simulink model "rev1BB"  (R2021a)
settings: Solver=FixedStepAuto  StartTime=0.0  StopTime=((((preLen+100+dataLenSymbols)*1+pad_first*3)*basePer))*2.5  RelTol=1e-3
values from neighbouring files (symbols this model uses):
  agcDesired = 0    [rev1BB_setup.m]
  agcStep = 2^-8    (= 0.00390625)    [rev1BB_setup.m]
  awgnSeed = abs(dBSnrRange(dBSnrInd)*1000+trial+10000000)    [plotBer.m]    (also in plotBerParSim.m; rev1BB_startup.m = 67)
  basePer = 1/baseFreq    (= 5e-08)    [rev1BB_setup.m]
  bitsPerSymbolHeader = log2(radixHeader)    [rev1BB_setup.m]
  bitsPerSymbolMax = log2(radixMax)    [rev1BB_setup.m]
  cefEarlyWarning = 256    [rev1BB_setup.m]
  cefLen = length(x_CEF)    [rev1BB_setup.m]
  cfoNcoWordLen = 16    [rev1BB_setup.m]
  channelFIR = zeros(1, round(maxSampleDelay)+1)    [rev1BB_simParams_setup.m]
  corr_peak_exclude_trigger = 1+corr_peak_trigger    (= 1.4)    [rev1BB_setup.m]
  corr_peak_trigger = 0.40    (= 0.4)    [rev1BB_setup.m]
  cr_i = 0.020    (= 0.02)    [rev1BB_setup.m]
  cr_i_preamp = 2^-9    (= 0.001953125)    [rev1BB_setup.m]
  cr_p = 0.015    [rev1BB_setup.m]
  dataLenSymbols = header_len_bytes*8/bitsPerSymbolHeader + frame_len_bytes*8/bitsPerSymbol    [rev1BB_setup.m]
  enableTRFreqCorrection = true    [rev1BB_setup.m]
  freeze_agc_in_CEF = true    [rev1BB_setup.m]
  freeze_agc_in_HeaderPayload = true    [rev1BB_setup.m]
  freeze_fineCFO_in_CEF = false    [rev1BB_setup.m]
  freeze_fineCFO_in_HeaderPayload = false    [rev1BB_setup.m]
  golay_type = golayType    (= 32)    [rev1BB_setup.m]
  golayType = 32    [rev1BB_setup.m]
  lmsEqDepth = 16    [rev1BB_setup.m]
  lmsStep_meta = (lmsStep_final - lmsStep_init)/cefLen    [rev1BB_setup.m]
  manChan = false    [rev1BB_simParams_setup.m]
  minSTFPeaks = 3    [rev1BB_setup.m]
  modBPS = [1, 2, 4]    [rev1BB_setup.m]
  modKeys = [0, 1, 2]    [rev1BB_setup.m]
  overSample = 3    [berCurve.m]    (also in rev1BB_setup.m = 4)
  qam16_demod_scale_factor = qam16_hdl_distance/qam16_power_normalized_distance    [rev1BB_setup.m]
  rcRxFilt = rcSqrtFilt    [rev1BB_setup.m]
  rcTxFilt = rcSqrtFilt    [rev1BB_setup.m]
  RxAGCCorrectionLoopPartition = 3    [rev1BB_setup.m]
  RxAGCPwrAvgPartition = 2    [rev1BB_setup.m]
  RxCoarseCFOPartition = 13    [rev1BB_setup.m]
  RxDemodPartition = 15    [rev1BB_setup.m]
  RxEQPartition = 14    [rev1BB_setup.m]
  RxFeedbackPipelining = 64*16    (= 1024)    [rev1BB_setup.m]
  RxFineCFOPartition = 15    [rev1BB_setup.m]
  RxFreezeControllerPartition = 17    [rev1BB_setup.m]
  RxFreezeFeedbackPipelining = RxFeedbackPipelining    (= 1024)    [rev1BB_setup.m]
  RxHeaderDemodPartition = 15    [rev1BB_setup.m]
  RxHeaderParsePartition = 15    [rev1BB_setup.m]
  RxPackerPartition = 16    [rev1BB_setup.m]
  RxPacketControllerPartition = 17    [rev1BB_setup.m]
  RxRRCPartition = 1    [rev1BB_setup.m]
  RxTimingRecoveryControlPartition = 8    [rev1BB_setup.m]
  RxTimingRecoveryDelayAccumPartition = 10    [rev1BB_setup.m]
  RxTimingRecoveryEarlyLatePartition = 10    [rev1BB_setup.m]
  RxTimingRecoveryFreqEstPartition = 10    [rev1BB_setup.m]
  RxTimingRecoveryGolayCorrelatorPartition = 6    [rev1BB_setup.m]
  RxTimingRecoveryGolayPeakDetectPartition = 7    [rev1BB_setup.m]
  RxTimingRecoverySymbolClockPartition = 9    [rev1BB_setup.m]
  RxTimingRecoveryVariableDelayPartition = 5    [rev1BB_setup.m]
  timing_cefEarlyWarningTollerance = 5    [rev1BB_setup.m]
  timing_correlator_pipeline = 1    [rev1BB_setup.m]
  timing_differentiator_grpDelay_roundUp = ceil((timing_differentiator_len)/2+timing_differentiator_pipeline)    [rev1BB_setup.m]
  timing_differentiator_pipeline = 1    [rev1BB_setup.m]
  timing_p = -0.215    [rev1BB_setup.m]
  timing_tolerance = 4    [rev1BB_setup.m]
  timingDifferentiatorFilt = timingDifferentiatorFiltObj.Coefficients    [rev1BB_setup.m]
  timingMaxSymbols = dataLenSymbols + length(x_CEF) + length(x_STF)/x_STFRepCount*2+100    [rev1BB_setup.m]
  timingRecoveryDoneSamplesEarly = floor(RxFeedbackPipelining/overSample) - delayToOutputFromDataFSM-1    [rev1BB_setup.m]
  timingRecoveryFreqCorrectionAvgLen = 32    [rev1BB_setup.m]
  timingRecoveryFreqCorrectionDiscardLastN = 2    [rev1BB_setup.m]
  trEarlyLateIGain = -0.000000050    (= -5e-08)    [rev1BB_setup.m]
  trEarlyLatePGain = -0.00225    [rev1BB_setup.m]
  trFarrowTaps = 4    [rev1BB_setup.m]
  trFeedbackPipelining = 64*8    (= 512)    [rev1BB_setup.m]
  trIntPhaseCounterInit = mod(timing_differentiator_grpDelay_roundUp, overSample)    [rev1BB_setup.m]
  trMatch = mod(-trLenToFSM, overSample)    [rev1BB_setup.m]
  trTappedDelayLen = trTappedDelayBase+trFarrowTaps    (= 44)    [rev1BB_setup.m]
  tx_rx_gain = 1    [rev1BB_simParams_setup.m]
  TxResampleModulatorPartition = 1    [rev1BB_setup.m]
  TxRRCFilterPartition = 2    [rev1BB_setup.m]
  txTimingOffset = 0    [plotBer.m]    (also in plotBerParSim.m; rev1BB_startup.m = 2e-05)
  txTimingPhase = channelizerUpDownSampling*overSample*4+1    [rev1BB_simParams_setup.m]
  x_CEF = xSpectrum_CEF_short    [rev1BB_setup.m]
  x_STFRepCount = nSpectrum_STFRepCount_short    (= 60)    [rev1BB_setup.m]
undefined symbols (not defined in the file or in its folder): doppler, magnitude
libraries: simulink x29, rev1CyclopsLib x20, commdigbbndpm3 x9, dspsigops x6, commdigbbndam3 x4, hdlsllib x2, commchan3 x2, commrflib2 x1
(part 1 of 3)
settings Model: Creator=cyarp  LastModifiedBy=cyarp
settings SolverCC: AlgebraicLoopSolver=TrustRegion
settings OptimizationCC: SimCompilerOptimization=on
settings DebuggingCC: SFMachineParentedDataDiag=warning
settings SFSimCC: SimHardwareAcceleration=native

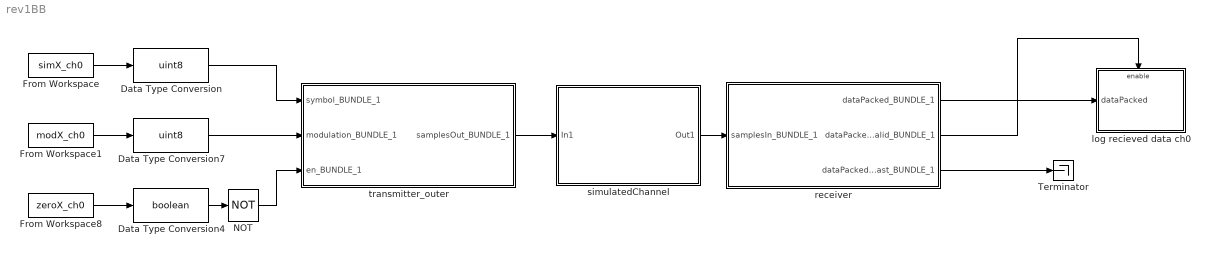
== system rev1BB ==
  Data Type Conversion : DataTypeConversion  OutDataTypeStr=uint8  RndMeth=Nearest
  Data Type Conversion4 : DataTypeConversion  OutDataTypeStr=boolean  RndMeth=Nearest
  Data Type Conversion7 : DataTypeConversion  OutDataTypeStr=uint8  RndMeth=Nearest
  From Workspace : FromWorkspace  VariableName=simX_ch0  SampleTime=basePer*1  Interpolate=off  OutputAfterFinalValue=Setting to zero
  From Workspace1 : FromWorkspace  VariableName=modX_ch0  SampleTime=basePer*1  Interpolate=off  OutputAfterFinalValue=Setting to zero
  From Workspace8 : FromWorkspace  VariableName=zeroX_ch0  SampleTime=basePer*1  Interpolate=off  OutputAfterFinalValue=Setting to zero
  NOT : Logic  Operator=NOT  IconShape=distinctive  AllPortsSameDT=off  OutDataTypeStr=boolean
  Terminator : Terminator
  log recieved data ch0 : Subsystem
  receiver : Subsystem
  simulatedChannel : Subsystem
  transmitter_outer : Subsystem
  wires:
  From Workspace/1 -> Data Type Conversion/1
  From Workspace1/1 -> Data Type Conversion7/1
  From Workspace8/1 -> Data Type Conversion4/1
  Data Type Conversion4/1 -> NOT/1
  simulatedChannel/1(Out1) -> receiver/1(samplesIn_BUNDLE_1)
  receiver/1(dataPacked_BUNDLE_1) -> log recieved data ch0/1(dataPacked)
  receiver/2(dataPackedValid_BUNDLE_1) -> log recieved data ch0/Enable
  receiver/3(dataPackedLast_BUNDLE_1) -> Terminator/1
  Data Type Conversion/1 -> transmitter_outer/1(symbol_BUNDLE_1)
  Data Type Conversion7/1 -> transmitter_outer/2(modulation_BUNDLE_1)
  NOT/1 -> transmitter_outer/3(en_BUNDLE_1)
  transmitter_outer/1(samplesOut_BUNDLE_1) -> simulatedChannel/1(In1)

== system rev1BB/log recieved data ch0 ==
  dataPacked : Inport
  Enable : EnablePort
  To Workspace1 : ToWorkspace  VariableName=data_recieved_packed_ch0  SampleTime=-1
      settings: Save2DSignal=2-D array (concatenate along first dimension)
  wires:
  dataPacked/1 -> To Workspace1/1

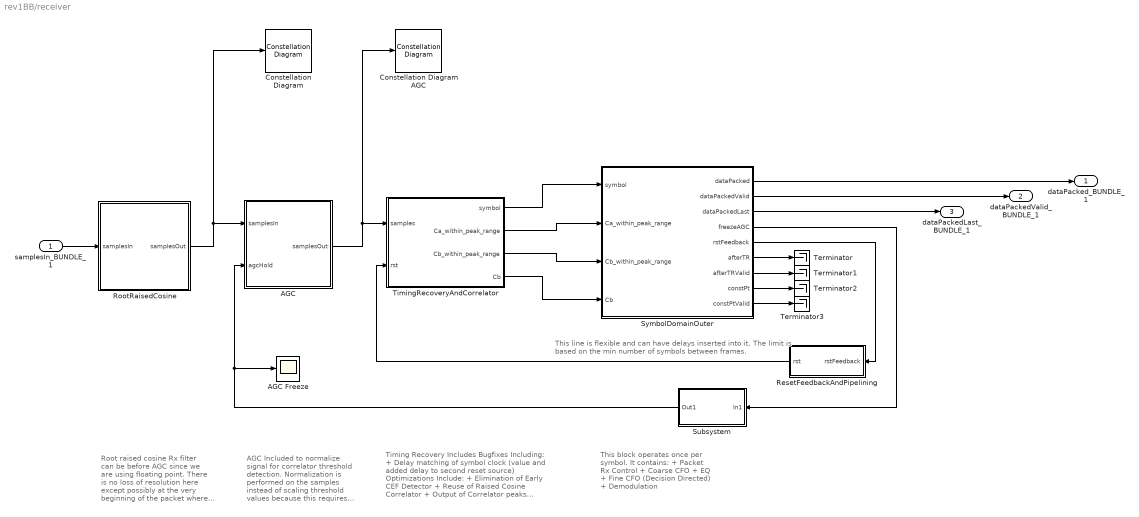
== system rev1BB/receiver ==
  note: This line is flexible and can have delays inserted into it.
      | The limit is based on the min number of symbols between frames.
  note: Timing Recovery Includes Bugfixes Including:
      | + Delay matching of symbol clock (value and added delay
      | to second reset source)
      |
      | Optimizations Include:
      | + Elimination of Early CEF Detector
      | + Reuse of Raised Cosine Correlator
      | + Output of Correlator peaks aligned with symbols
  note: This block operates once per symbol.
      |
      | It contains:
      | + Packet Rx Control
      | + Coarse CFO
      | + EQ
      | + Fine CFO (Decision Directed)
      | + Demodulation
  note: AGC Included to normalize signal for correlator threshold detection.  Normalization is performed on the samples instead of scaling threshold values because this requires fewer operations (once per sample instead of once per sample per threshold detector)
      |
      | This was also modified so that freezing the AGC stops power estimation.
  note: Root raised cosine Rx filter can be before AGC since we are using floating point. There is no loss of resolution here except possibly at the very beginning of the packet where a high power signal will show up.
  samplesIn_BUNDLE_1 : Inport
  AGC : Subsystem
  AGC Freeze : Scope
  Constellation Diagram : ConstellationDiagram
  Constellation Diagram AGC : ConstellationDiagram
  ResetFeedbackAndPipelining : Subsystem
  RootRaisedCosine : Subsystem
  Subsystem : Subsystem
  SymbolDomainOuter : Subsystem
  Terminator{,1..3} (4 alike) : Terminator
  TimingRecoveryAndCorrelator : Subsystem
  dataPacked_BUNDLE_1 : Outport
  dataPackedValid_BUNDLE_1 : Outport  Port=2
  dataPackedLast_BUNDLE_1 : Outport  Port=3
  wires:
  samplesIn_BUNDLE_1/1 -> RootRaisedCosine/1(samplesIn)
  AGC/1(samplesOut) -> Constellation Diagram AGC/1, TimingRecoveryAndCorrelator/1(samples)
  RootRaisedCosine/1(samplesOut) -> Constellation Diagram/1, AGC/1(samplesIn)
  ResetFeedbackAndPipelining/1(rst) -> TimingRecoveryAndCorrelator/2(rst)
  Subsystem/1(Out1) -> AGC Freeze/1, AGC/2(agcHold)
  TimingRecoveryAndCorrelator/1(symbol) -> SymbolDomainOuter/1(symbol)
  TimingRecoveryAndCorrelator/2(Ca_within_peak_range) -> SymbolDomainOuter/2(Ca_within_peak_range)
  TimingRecoveryAndCorrelator/3(Cb_within_peak_range) -> SymbolDomainOuter/3(Cb_within_peak_range)
  TimingRecoveryAndCorrelator/4(Cb) -> SymbolDomainOuter/4(Cb)
  SymbolDomainOuter/1(dataPacked) -> dataPacked_BUNDLE_1/1
  SymbolDomainOuter/2(dataPackedValid) -> dataPackedValid_BUNDLE_1/1
  SymbolDomainOuter/3(dataPackedLast) -> dataPackedLast_BUNDLE_1/1
  SymbolDomainOuter/4(freezeAGC) -> Subsystem/1(In1)
  SymbolDomainOuter/5(rstFeedback) -> ResetFeedbackAndPipelining/1(rstFeedback)
  SymbolDomainOuter/6(afterTR) -> Terminator/1
  SymbolDomainOuter/7(afterTRValid) -> Terminator1/1
  SymbolDomainOuter/8(constPt) -> Terminator2/1
  SymbolDomainOuter/9(constPtValid) -> Terminator3/1

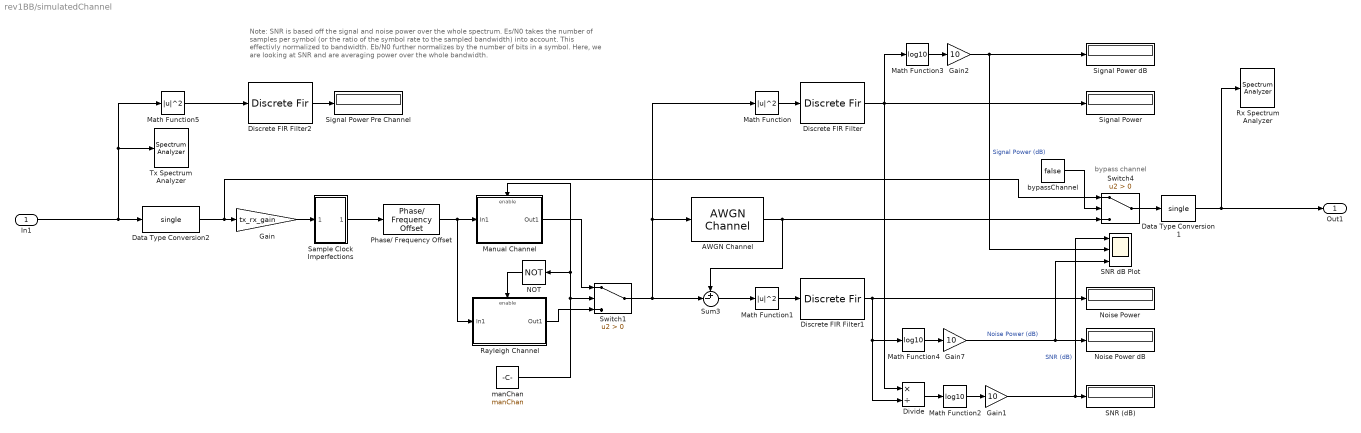
== system rev1BB/simulatedChannel ==
  note: Note: SNR is based off the signal and noise power over the whole spectrum.
      | Es/N0 takes the number of samples per symbol (or the ratio of the symbol rate to the sampled bandwidth) into account.  This effectivly normalized to bandwidth.
      | Eb/N0 further normalizes by the number of bits in a symbol.
      |
      | Here, we are looking at SNR and are averaging power over the whole bandwidth.
  note: bypass channel
  In1 : Inport
  AWGN Channel : commchan3/AWGN Channel  InputProcessing=Columns as channels (frame based)  seed=awgnSeed  noiseMode="Signal to noise ratio  (SNR)"  EbNodB=awgnEbN0  EsNodB=10  SNRdB=awgnSNR  bitsPerSym=1  Ps=1  Tsym=basePer  variance=1
  Data Type Conversion1 : DataTypeConversion  OutDataTypeStr=single
  Data Type Conversion2 : DataTypeConversion  OutDataTypeStr=single
  Discrete FIR Filter : DiscreteFir  Coefficients=ones(1,10000)./10000  InputProcessing=Columns as channels (frame based)
  Discrete FIR Filter1 : DiscreteFir  Coefficients=ones(1,10000)./10000  InputProcessing=Columns as channels (frame based)
  Discrete FIR Filter2 : DiscreteFir  Coefficients=ones(1,10000)./10000  InputProcessing=Columns as channels (frame based)
  Divide : Product  Inputs=*/
  Gain : Gain  Gain=tx_rx_gain
  Gain1 : Gain  Gain=10
  Gain2 : Gain  Gain=10
  Gain7 : Gain  Gain=10
  Manual Channel : Subsystem
  Math Function : Math  Operator=magnitude^2  SignedPower=on  OutputSignalType=real  SaturateOnIntegerOverflow=on
  Math Function1 : Math  Operator=magnitude^2  SignedPower=on  OutputSignalType=real  SaturateOnIntegerOverflow=on
  Math Function2 : Math  Operator=log10  SignedPower=on  OutputSignalType=real  SaturateOnIntegerOverflow=on
  Math Function3 : Math  Operator=log10  SignedPower=on  OutputSignalType=real  SaturateOnIntegerOverflow=on
  Math Function4 : Math  Operator=log10  SignedPower=on  OutputSignalType=real  SaturateOnIntegerOverflow=on
  Math Function5 : Math  Operator=magnitude^2  SignedPower=on  OutputSignalType=real  SaturateOnIntegerOverflow=on
  NOT : Logic  Operator=NOT  IconShape=distinctive  AllPortsSameDT=off  OutDataTypeStr=boolean
  Noise Power : Display
  Noise Power dB : Display
  Phase/ Frequency Offset : commrflib2/Phase// Frequency Offset  phaseOffset=rxPhaseOffset  freqPort=off  freqOffset=freqOffsetHz
  Rayleigh Channel : Subsystem
  Rx Spectrum Analyzer : SpectrumAnalyzer
  SNR (dB) : Display
  SNR dB Plot : Scope  NumInputPorts=3
  Sample Clock Imperfections : Subsystem
  Signal Power : Display
  Signal Power Pre Channel : Display
  Signal Power dB : Display
  Sum3 : Sum  Inputs=+-|
  Switch1 : Switch  Criteria=u2 > Threshold
  Switch4 : Switch  Criteria=u2 > Threshold
  Tx Spectrum Analyzer : SpectrumAnalyzer
  bypassChannel : Constant  Value=false  OutDataTypeStr=boolean
  manChan : Constant  Value=manChan  OutDataTypeStr=boolean
  Out1 : Outport
  wires:
  Data Type Conversion2/1 -> Switch4/1, Gain/1
  Sample Clock Imperfections/1(Out1) -> Phase/ Frequency Offset/1
  Data Type Conversion1/1 -> Out1/1, Rx Spectrum Analyzer/1
  bypassChannel/1 -> Switch4/2
  Gain2/1 -> SNR dB Plot/2, Signal Power dB/1  "Signal Power (dB)"
  AWGN Channel/1 -> Switch4/3, Sum3/1
  Gain/1 -> Sample Clock Imperfections/1(In1)
  Math Function/1 -> Discrete FIR Filter/1
  Sum3/1 -> Math Function1/1
  Switch1/1 -> Math Function/1, AWGN Channel/1, Sum3/2
  Math Function3/1 -> Gain2/1
  Gain7/1 -> SNR dB Plot/3, Noise Power dB/1  "Noise Power (dB)"
  Switch4/1 -> Data Type Conversion1/1
  Divide/1 -> Math Function2/1
  Gain1/1 -> SNR dB Plot/1, SNR (dB)/1  "SNR (dB)"
  Math Function2/1 -> Gain1/1
  Discrete FIR Filter/1 -> Math Function3/1, Divide/1, Signal Power/1
  Math Function4/1 -> Gain7/1
  Phase/ Frequency Offset/1 -> Manual Channel/1(In1), Rayleigh Channel/1(In1)
  Discrete FIR Filter1/1 -> Math Function4/1, Divide/2, Noise Power/1
  Math Function1/1 -> Discrete FIR Filter1/1
  In1/1 -> Math Function5/1, Tx Spectrum Analyzer/1, Data Type Conversion2/1
  Math Function5/1 -> Discrete FIR Filter2/1
  Discrete FIR Filter2/1 -> Signal Power Pre Channel/1
  manChan/1 -> Switch1/2, Manual Channel/Enable, NOT/1
  Rayleigh Channel/1(Out1) -> Switch1/3
  Manual Channel/1(Out1) -> Switch1/1
  NOT/1 -> Rayleigh Channel/Enable

== system rev1BB/transmitter_outer ==
  symbol_BUNDLE_1 : Inport
  modulation_BUNDLE_1 : Inport  Port=2
  en_BUNDLE_1 : Inport  Port=3
  transmitter : Subsystem
  samplesOut_BUNDLE_1 : Outport
  wires:
  transmitter/1(samplesOut) -> samplesOut_BUNDLE_1/1
  modulation_BUNDLE_1/1 -> transmitter/2(modulation)
  symbol_BUNDLE_1/1 -> transmitter/1(symbol)
  en_BUNDLE_1/1 -> transmitter/3(en)

== system rev1BB/receiver/AGC ==
  note: Note, the enabled subsystem was split because lazy FIFO evaluation
      | is not yet implemented in Laminar.  Because the enabled subsystems are all
      | driven by a common source and no state was placed between them,
      | the result should be the same.  Enabled subsystem is passed through the local
      | pipelines of partitions to hopefully capaitalize on communication locality
      | among these partitions (assuming these will be placed in the same L3).  Involves
      | using a dummy node to pass the enable signal in AGCLoopAndCorrect.
      |
      | Note that this arragment will cause one element to be in the sample FIFO into
      | AGCLoopAndCorrect at all times because of the dependence on AGC Pwr Avg
      |
      | ---
      | Change: Now forwarding samples from AGC Pwr Avg to AGCLoopAndCorrect.
  samplesIn : Inport
  agcHold : Inport  Port=2
  AGCLoopAndCorrect : Subsystem
  AGCPwrAvg : Subsystem
  Terminator : Terminator
  Terminator1 : Terminator
  samplesOut : Outport
  wires:
  samplesIn/1 -> AGCPwrAvg/1(samples)
  agcHold/1 -> AGCPwrAvg/2(freeze)
  AGCPwrAvg/2(lnPwrAvg) -> AGCLoopAndCorrect/2(pwrAvg)
  AGCPwrAvg/3(en) -> AGCLoopAndCorrect/3(enable)
  AGCLoopAndCorrect/1(samplesOut) -> samplesOut/1
  AGCPwrAvg/1(samplesOut) -> AGCLoopAndCorrect/1(samplesIn)
  AGCLoopAndCorrect/2(lnPwr) -> Terminator/1
  AGCLoopAndCorrect/3(en) -> Terminator1/1

== system rev1BB/receiver/ResetFeedbackAndPipelining ==
  rstFeedback : Inport
  BinaryPosEdgeDetect : rev1CyclopsLib/BinaryPosEdgeDetect  SystemSampleTime=-1  VariantActivationTime=update diagram  Latency=0  AutoFrameSizeCalculation=off
  Delay : Delay  DelayLength=RxFeedbackPipelining  UseCircularBuffer=on
  Terminator2 : Terminator
  VITIS_PARTITION : Constant  Value=RxTimingRecoveryControlPartition
  rst : Outport
  wires:
  rstFeedback/1 -> Delay/1
  BinaryPosEdgeDetect/1 -> rst/1
  Delay/1 -> BinaryPosEdgeDetect/1
  VITIS_PARTITION/1 -> Terminator2/1

== system rev1BB/receiver/RootRaisedCosine ==
  samplesIn : Inport
  Terminator2 : Terminator
  VITIS_PARTITION : Constant  Value=RxRRCPartition
  rootRaisedCosineFilter : DiscreteFir  Coefficients=rcRxFilt
  samplesOut : Outport
  wires:
  rootRaisedCosineFilter/1 -> samplesOut/1
  VITIS_PARTITION/1 -> Terminator2/1
  samplesIn/1 -> rootRaisedCosineFilter/1

== system rev1BB/receiver/Subsystem ==
  In1 : Inport
  Delay : Delay  DelayLength=RxFreezeFeedbackPipelining  UseCircularBuffer=on
  Terminator2 : Terminator
  VITIS_PARTITION : Constant  Value=RxAGCPwrAvgPartition
  Out1 : Outport
  wires:
  In1/1 -> Delay/1
  Delay/1 -> Out1/1
  VITIS_PARTITION/1 -> Terminator2/1

== system rev1BB/receiver/SymbolDomainOuter ==
  symbol : Inport
  Ca_within_peak_range : Inport  Port=2
  Cb_within_peak_range : Inport  Port=3
  Cb : Inport  Port=4
  Terminator2 : Terminator
  VITIS_CLOCK_DOMAIN_SymbolDomain : Subsystem
  VITIS_PARTITION : Constant  Value=RxPacketControllerPartition
  dataPacked : Outport
  dataPackedValid : Outport  Port=2
  dataPackedLast : Outport  Port=3
  freezeAGC : Outport  Port=4
  rstFeedback : Outport  Port=5
  afterTR : Outport  Port=6
  afterTRValid : Outport  Port=7
  constPt : Outport  Port=8
  constPtValid : Outport  Port=9
  wires:
  VITIS_CLOCK_DOMAIN_SymbolDomain/6(afterTR) -> afterTR/1
  VITIS_CLOCK_DOMAIN_SymbolDomain/3(dataPackedLast) -> dataPackedLast/1
  VITIS_CLOCK_DOMAIN_SymbolDomain/1(dataPacked) -> dataPacked/1
  VITIS_CLOCK_DOMAIN_SymbolDomain/2(dataPackedValid) -> dataPackedValid/1
  Cb_within_peak_range/1 -> VITIS_CLOCK_DOMAIN_SymbolDomain/3(Cb_within_peak_range)
  VITIS_CLOCK_DOMAIN_SymbolDomain/5(rstFeedback) -> rstFeedback/1
  VITIS_CLOCK_DOMAIN_SymbolDomain/4(freezeAGC) -> freezeAGC/1
  VITIS_CLOCK_DOMAIN_SymbolDomain/9(constPtValid) -> constPtValid/1
  VITIS_CLOCK_DOMAIN_SymbolDomain/7(afterTRValid) -> afterTRValid/1
  VITIS_CLOCK_DOMAIN_SymbolDomain/8(constPt) -> constPt/1
  symbol/1 -> VITIS_CLOCK_DOMAIN_SymbolDomain/1(symbol)
  Cb/1 -> VITIS_CLOCK_DOMAIN_SymbolDomain/4(Cb)
  Ca_within_peak_range/1 -> VITIS_CLOCK_DOMAIN_SymbolDomain/2(Ca_within_peak_range)
  VITIS_PARTITION/1 -> Terminator2/1

== system rev1BB/receiver/TimingRecoveryAndCorrelator ==
  note: Because of the loop and the forks from earlier partitions to partitions further in the loops, there will be FIFOs with values always present. Make sure the FIFOs are sized to accomodate this.
  samples : Inport
  rst : Inport  Port=2
  EarlyLate : Subsystem
  FreqEstDelayAccumulator : Subsystem
  GolayPeakDetect : Subsystem
  GolayPeakDetectDecimSync : Subsystem
  SymbolClockOuter : Subsystem
  TRControl : Subsystem
  TimingDecimPhase : Scope
  VarDelayDecimSync : Subsystem
  VarDelayWithSampleAlignment : Subsystem
  symbol : Outport
  Ca_within_peak_range : Outport  Port=2
  Cb_within_peak_range : Outport  Port=3
  Cb : Outport  Port=4
  wires:
  GolayPeakDetect/1(Ca_within_peak_range) -> GolayPeakDetectDecimSync/1(In1), TRControl/1(cef_start)
  FreqEstDelayAccumulator/1(fullDelay) -> VarDelayWithSampleAlignment/2(delay)
  samples/1 -> VarDelayWithSampleAlignment/1(samples)
  GolayPeakDetect/4(Cb_phase_imbal) -> FreqEstDelayAccumulator/1(estimatedPhaseImbal)
  EarlyLate/1(earlyLateEstimate) -> FreqEstDelayAccumulator/6(earlyLateCorrection)
  SymbolClockOuter/1(symbolClockPrePhaseCorrection) -> EarlyLate/2(symbolClk)
  TRControl/6(trEstDone) -> FreqEstDelayAccumulator/5(stfDone), EarlyLate/4(trEstDone)
  TRControl/4(estimateNow) -> FreqEstDelayAccumulator/4(estimateNow), SymbolClockOuter/4(newPeriodAvail)
  TRControl/3(rstIntegerPhase) -> SymbolClockOuter/3(rst), FreqEstDelayAccumulator/3(rst)
  TRControl/5(trEstDoneEdge) -> FreqEstDelayAccumulator/2(trEstDoneEdge), EarlyLate/5(trEstDoneEdge), EarlyLate/3(rst)
  GolayPeakDetect/3(Cb_fine_peak_detect) -> TRControl/2(peak)
  rst/1 -> TRControl/3(rst)
  TRControl/1(receiving) -> SymbolClockOuter/1(recieving)
  TRControl/2(lastPeriod) -> SymbolClockOuter/2(lastGolayPeriod)
  VarDelayWithSampleAlignment/1(out) -> EarlyLate/1(pulseShapedCorr), GolayPeakDetect/1(In1)
  SymbolClockOuter/2(symbolPhase) -> GolayPeakDetectDecimSync/4(idx), TimingDecimPhase/1, VarDelayDecimSync/1(idx)
  GolayPeakDetect/2(Cb_within_peak_range) -> GolayPeakDetectDecimSync/2(In2)
  GolayPeakDetectDecimSync/1(Out1) -> Ca_within_peak_range/1
  GolayPeakDetectDecimSync/2(Out2) -> Cb_within_peak_range/1
  VarDelayWithSampleAlignment/2(Out2) -> VarDelayDecimSync/2(In2)
  VarDelayDecimSync/1(Out1) -> symbol/1
  GolayPeakDetect/5(Cb) -> GolayPeakDetectDecimSync/3(Cb)
  GolayPeakDetectDecimSync/3(Out3) -> Cb/1

== system rev1BB/simulatedChannel/Manual Channel ==
  In1 : Inport
  Enable : EnablePort
  Manual Channel : DiscreteFir  Coefficients=channelFIR  InputProcessing=Columns as channels (frame based)
  Out1 : Outport
  wires:
  In1/1 -> Manual Channel/1
  Manual Channel/1 -> Out1/1

== system rev1BB/simulatedChannel/Rayleigh Channel ==
  In1 : Inport
  Enable : EnablePort
  SISO Fading Channel : commchan3/SISO Fading Channel  InheritSampleRate=on  SampleRate=1  PathDelays=chanDelays  AveragePathGains=chanAvgPathGainsdB  NormalizePathGains=on  FadingDistribution=Rayleigh  KFactor=3  DirectPathDopplerShift=0  DirectPathInitialPhase=0  MaximumDopplerShift=maxDopplerHz  DopplerSpectrum=doppler('Jakes')  RandomStream=mt19937ar with seed  Seed=awgnSeed  PathGainsOutputPort=off  ChannelFilterDelayOutputPort=off  SimulateUsing=Interpreted execution  Visualization=Off  PathsForDopplerDisplay=1  SamplesToDisplay=25%
  Out1 : Outport
  wires:
  SISO Fading Channel/1 -> Out1/1
  In1/1 -> SISO Fading Channel/1

== system rev1BB/simulatedChannel/Sample Clock Imperfections ==
  note: Had to switch to FIR interpolate over Farrow because Farrow was resulting in some attenuation
      | at high frequencies which was problamatic for channelizing
  In1 : Inport
  Constant : Constant  Value=txTimingOffset  OutDataTypeStr=Inherit: Inherit via back propagation
  Delay : Delay  DelayLength=1  InitialCondition=txTimingPhase
  SampleClockDelay : Scope
  Sum : Sum  Inputs=|++
  Variable Fractional Delay : dspsigops/Variable Fractional Delay  mode=OBSOLETE  modeActive=FIR  L=20  FarrowL=40  R=80  alpha=1  dmax=1000  InputProcessing=Columns as channels (frame based)  ic=0  noDFT=off  fallbackFIR=Clip to the minimum value necessary for centered kernel  fallbackFarrow=Clip to the minimum value necessary for centered kernel  roundingMode=Zero  overflowMode=off
      settings: SourceProductBaseCode=DS
  Out1 : Outport  VectorParamsAs1DForOutWhenUnconnected=off
  wires:
  In1/1 -> Variable Fractional Delay/1
  Variable Fractional Delay/1 -> Out1/1
  Constant/1 -> Sum/1
  Sum/1 -> Delay/1
  Delay/1 -> Sum/2, SampleClockDelay/1, Variable Fractional Delay/2

== system rev1BB/transmitter_outer/transmitter ==
  symbol : Inport
  modulation : Inport  Port=2
  en : Inport  Port=3
  Constant : Constant  Value=0  OutDataTypeStr=Inherit: Inherit via back propagation  SampleTime=-1
  Constant1 : Constant  Value=0  OutDataTypeStr=Inherit: Inherit via back propagation  SampleTime=-1
  Real-Imag to Complex : RealImagToComplex
  Terminator2 : Terminator
  VITIS_CLOCK_DOMAIN_modulate : Subsystem
  VITIS_PARTITION : Constant  Value=TxResampleModulatorPartition
  enableSwitch : Switch  Criteria=u2 ~= 0
  rootRaisedCosineAndScale : Subsystem
  samplesOut : Outport
  wires:
  VITIS_PARTITION/1 -> Terminator2/1
  symbol/1 -> VITIS_CLOCK_DOMAIN_modulate/1(symbol)
  modulation/1 -> VITIS_CLOCK_DOMAIN_modulate/2(modulation)
  en/1 -> VITIS_CLOCK_DOMAIN_modulate/3(en)
  Constant1/1 -> Real-Imag to Complex/2
  Constant/1 -> Real-Imag to Complex/1
  VITIS_CLOCK_DOMAIN_modulate/2(enUpsampled) -> enableSwitch/2
  Real-Imag to Complex/1 -> enableSwitch/3
  enableSwitch/1 -> rootRaisedCosineAndScale/1(In1)
  rootRaisedCosineAndScale/1(Out1) -> samplesOut/1
  VITIS_CLOCK_DOMAIN_modulate/1(symbolUpsampled) -> enableSwitch/1

== system rev1BB/receiver/AGC/AGCLoopAndCorrect ==
  samplesIn : Inport
  pwrAvg : Inport  Port=2
  enable : Inport  Port=3
  AGCCorrectionLoopEnabled : Subsystem
  Product : Product  OutDataTypeStr=Inherit: Same as first input
  Terminator2 : Terminator
  VITIS_PARTITION : Constant  Value=RxAGCCorrectionLoopPartition
  agcCorrection : Scope
  samplesOut : Outport
  lnPwr : Outport  Port=2
  en : Outport  Port=3
  wires:
  samplesIn/1 -> Product/1
  Product/1 -> samplesOut/1
  AGCCorrectionLoopEnabled/1(correction) -> Product/2, agcCorrection/1
  VITIS_PARTITION/1 -> Terminator2/1
  pwrAvg/1 -> AGCCorrectionLoopEnabled/1(samples)
  AGCCorrectionLoopEnabled/2(lnPwr) -> lnPwr/1
  enable/1 -> en/1, AGCCorrectionLoopEnabled/Enable

== system rev1BB/receiver/AGC/AGCPwrAvg ==
  samples : Inport
  freeze : Inport  Port=2
  AGCPowerAvgEnabled : Subsystem
  NOT2 : Logic  Operator=NOT  IconShape=distinctive  AllPortsSameDT=off  OutDataTypeStr=boolean
  Terminator2 : Terminator
  VITIS_CONTEXT_ABSORB_BARRIER : Delay  DelayLength=0
  VITIS_PARTITION : Constant  Value=RxAGCPwrAvgPartition
  samplesOut : Outport
  lnPwrAvg : Outport  Port=2
  en : Outport  Port=3
  wires:
  freeze/1 -> NOT2/1
  samples/1 -> VITIS_CONTEXT_ABSORB_BARRIER/1
  VITIS_PARTITION/1 -> Terminator2/1
  VITIS_CONTEXT_ABSORB_BARRIER/1 -> samplesOut/1, AGCPowerAvgEnabled/1(samples)
  AGCPowerAvgEnabled/1(lnPwrAvg) -> lnPwrAvg/1
  NOT2/1 -> AGCPowerAvgEnabled/Enable, en/1

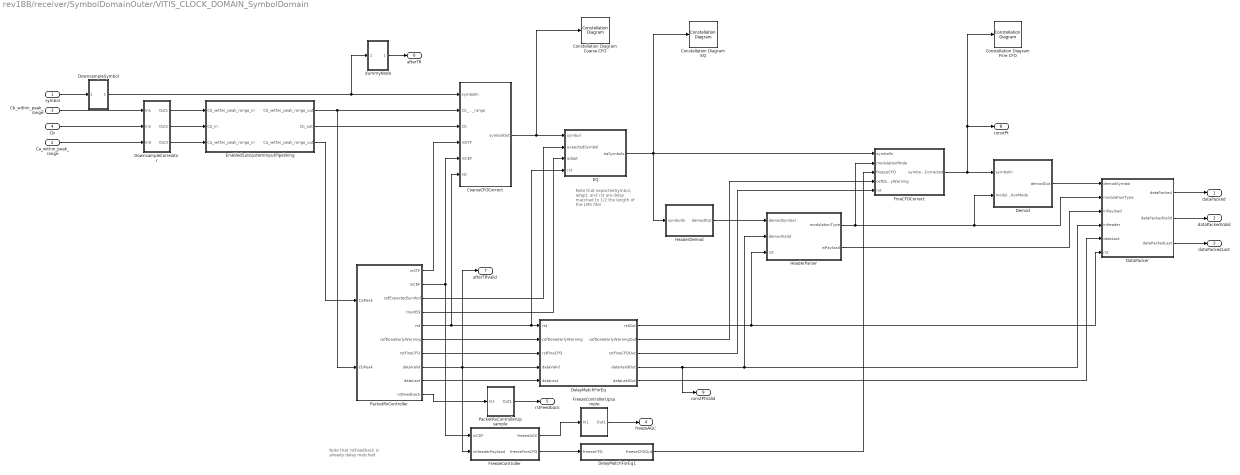
== system rev1BB/receiver/SymbolDomainOuter/VITIS_CLOCK_DOMAIN_SymbolDomain ==
  note: Note that rstFeedback is already delay matched
  note: Note that expectedSymbol, adapt, and rst are delay matched to 1/2 the length of the LMS fiter
  symbol : Inport
  Ca_within_peak_range : Inport  Port=2
  Cb_within_peak_range : Inport  Port=3
  Cb : Inport  Port=4
  CoarseCFOCorrect : Subsystem
  Constellation Diagram Coarse CFO : ConstellationDiagram
  Constellation Diagram EQ : ConstellationDiagram
  Constellation Diagram Fine CFO : ConstellationDiagram
  DataPacker : Subsystem
  DelayMatchForEq : Subsystem
  DelayMatchForEq1 : Subsystem
  Demod : Subsystem
  DownsampleCorrelator : Subsystem
  DownsampleSymbol : Subsystem
  EQ : Subsystem
  EnabledSubsystemInputPipelining : Subsystem
  FineCFOCorrect : Subsystem
  FreezeController : Subsystem
  FreezeControllerUpsample : Subsystem
  HeaderDemod : Subsystem
  HeaderParser : Subsystem
  PacketRxController : Subsystem
  PacketRxControllerUpsample : Subsystem
  dummyNode : Subsystem
  dataPacked : Outport
  dataPackedValid : Outport  Port=2
  dataPackedLast : Outport  Port=3
  freezeAGC : Outport  Port=4
  rstFeedback : Outport  Port=5
  afterTR : Outport  Port=6
  afterTRValid : Outport  Port=7
  constPt : Outport  Port=8
  constPtValid : Outport  Port=9
  wires:
  FineCFOCorrect/1(symbolCorrected) -> constPt/1, Constellation Diagram Fine CFO/1, Demod/1(symbolIn)
  Demod/1(demodOut) -> DataPacker/1(demodSymbol)
  CoarseCFOCorrect/1(symbolOut) -> Constellation Diagram Coarse CFO/1, EQ/1(symbol)
  EQ/1(eqSymbols) -> HeaderDemod/1(symbolIn), Constellation Diagram EQ/1, FineCFOCorrect/1(symbolIn)
  PacketRxController/1(inSTF) -> CoarseCFOCorrect/4(inSTF)
  PacketRxController/2(inCEF) -> FreezeController/1(inCEF), CoarseCFOCorrect/5(inCEF)
  PacketRxController/5(rst) -> DelayMatchForEq/1(rst), EQ/4(rst), CoarseCFOCorrect/6(rst)
  PacketRxController/4(trainEQ) -> EQ/3(adapt)
  PacketRxController/3(cefExpectedSymbol) -> EQ/2(expectedSymbol)
  DataPacker/1(dataPacked) -> dataPacked/1
  DataPacker/2(dataPackedValid) -> dataPackedValid/1
  DataPacker/3(dataPackedLast) -> dataPackedLast/1
  DelayMatchForEq/2(cefDoneEarlyWarningOut) -> FineCFOCorrect/4(cefDoneEarlyWarning)
  DelayMatchForEq/3(rstFineCFOOut) -> FineCFOCorrect/5(rst)
  PacketRxController/6(cefDoneEarlyWarning) -> DelayMatchForEq/2(cefDoneEarlyWarning)
  PacketRxController/7(rstFineCFO) -> DelayMatchForEq/3(rstFineCFO)
  PacketRxController/8(dataValid) -> afterTRValid/1, FreezeController/2(inHeaderPayload), DelayMatchForEq/4(dataValid)
  PacketRxController/9(dataLast) -> DelayMatchForEq/5(dataLast)
  DelayMatchForEq1/1(freezeCFOOut) -> FineCFOCorrect/3(freezeCFO)
  FreezeController/2(freezeFineCFO) -> DelayMatchForEq1/1(freezeCFO)
  DelayMatchForEq/1(rstOut) -> DataPacker/6(rst), HeaderParser/3(rst)
  HeaderParser/1(modulationType) -> DataPacker/2(modulationType), Demod/2(modulationMode), FineCFOCorrect/2(modulationMode)
  DelayMatchForEq/4(dataValidOut) -> HeaderParser/2(demodValid), DataPacker/4(inHeader), constPtValid/1
  HeaderParser/2(inPayload) -> DataPacker/3(inPayload)
  DelayMatchForEq/5(dataLastOut) -> DataPacker/5(dataLast)
  EnabledSubsystemInputPipelining/1(Cb_within_peak_range_out) -> PacketRxController/2(CbPeak), CoarseCFOCorrect/2(Cb_within_peak_range)
  EnabledSubsystemInputPipelining/2(Cb_out) -> CoarseCFOCorrect/3(Cb)
  EnabledSubsystemInputPipelining/3(Ca_within_peak_range_out) -> PacketRxController/1(CaPeak)
  dummyNode/1(Out1) -> afterTR/1
  Cb_within_peak_range/1 -> DownsampleCorrelator/1(In1)
  Cb/1 -> DownsampleCorrelator/2(In2)
  Ca_within_peak_range/1 -> DownsampleCorrelator/3(In3)
  DownsampleCorrelator/1(Out1) -> EnabledSubsystemInputPipelining/1(Cb_within_peak_range_in)
  DownsampleCorrelator/2(Out2) -> EnabledSubsystemInputPipelining/2(Cb_in)
  DownsampleCorrelator/3(Out3) -> EnabledSubsystemInputPipelining/3(Ca_within_peak_range_in)
  DownsampleSymbol/1(Out1) -> dummyNode/1(In1), CoarseCFOCorrect/1(symbolIn)
  symbol/1 -> DownsampleSymbol/1(In1)
  PacketRxController/10(rstFeedback) -> PacketRxControllerUpsample/1(In1)
  PacketRxControllerUpsample/1(Out1) -> rstFeedback/1
  FreezeController/1(freezeAGC) -> FreezeControllerUpsample/1(In1)
  FreezeControllerUpsample/1(Out1) -> freezeAGC/1
  HeaderDemod/1(demodOut) -> HeaderParser/1(demodSymbol)

== system rev1BB/receiver/TimingRecoveryAndCorrelator/EarlyLate ==
  pulseShapedCorr : Inport
  symbolClk : Inport  Port=2
  rst : Inport  Port=3
  trEstDone : Inport  Port=4
  trEstDoneEdge : Inport  Port=5
  EarlyLateEst : Subsystem
  OR2 : Logic  Operator=OR  IconShape=distinctive  AllPortsSameDT=off  OutDataTypeStr=boolean
  Terminator2 : Terminator
  VITIS_PARTITION : Constant  Value=RxTimingRecoveryEarlyLatePartition
  delayToBreakComboLoop1 : Delay  DelayLength=1
  earlyLateEstimate : Outport
  wires:
  delayToBreakComboLoop1/1 -> earlyLateEstimate/1
  EarlyLateEst/1(earlyLateCorrection) -> delayToBreakComboLoop1/1
  VITIS_PARTITION/1 -> Terminator2/1
  OR2/1 -> EarlyLateEst/Enable
  trEstDone/1 -> OR2/1
  trEstDoneEdge/1 -> OR2/2
  pulseShapedCorr/1 -> EarlyLateEst/1(pulseShapedCorr)
  symbolClk/1 -> EarlyLateEst/2(symbolClk)
  rst/1 -> EarlyLateEst/3(rst)

== system rev1BB/receiver/TimingRecoveryAndCorrelator/FreqEstDelayAccumulator ==
  estimatedPhaseImbal : Inport
  trEstDoneEdge : Inport  Port=2
  rst : Inport  Port=3
  estimateNow : Inport  Port=4
  stfDone : Inport  Port=5
  earlyLateCorrection : Inport  Port=6
  DelayAccum : Subsystem
  EstimateTimingFreqOffset : Subsystem  mask{avgOver=timingRecoveryFreqCorrectionAvgLen, numToClear=timingRecoveryFreqCorrectionDiscardLastN, scaleBy=(1/golay_type)*(1/overSample)}
      mask prompts: avgOver "Number of Measurements to Average Over"; numToClear "Number of Measurements to Clear"; scaleBy "Scale Output By"
  OR : Logic  Operator=OR  Inputs=3  IconShape=distinctive  AllPortsSameDT=off  OutDataTypeStr=boolean
  Terminator2 : Terminator
  VITIS_PARTITION : Constant  Value=RxTimingRecoveryFreqEstPartition
  timing_p : Gain  Gain=timing_p
  fullDelay : Outport
  wires:
  OR/1 -> EstimateTimingFreqOffset/Enable
  estimateNow/1 -> DelayAccum/4(proportionalCorrectionValid), OR/2
  estimatedPhaseImbal/1 -> timing_p/1
  VITIS_PARTITION/1 -> Terminator2/1
  EstimateTimingFreqOffset/1(avg) -> DelayAccum/2(freqEstimateCorrection)
  stfDone/1 -> DelayAccum/5(stfDone)
  earlyLateCorrection/1 -> DelayAccum/7(earlyLateCorrection)
  DelayAccum/1(fullDelay) -> fullDelay/1
  timing_p/1 -> DelayAccum/1(proportionalCorrectionDurringSTF), EstimateTimingFreqOffset/1(toAvg)
  trEstDoneEdge/1 -> EstimateTimingFreqOffset/2(clearLastN), OR/3, DelayAccum/3(trEstDoneEdge)
  rst/1 -> DelayAccum/6(rstDelay), OR/1, EstimateTimingFreqOffset/3(rst)

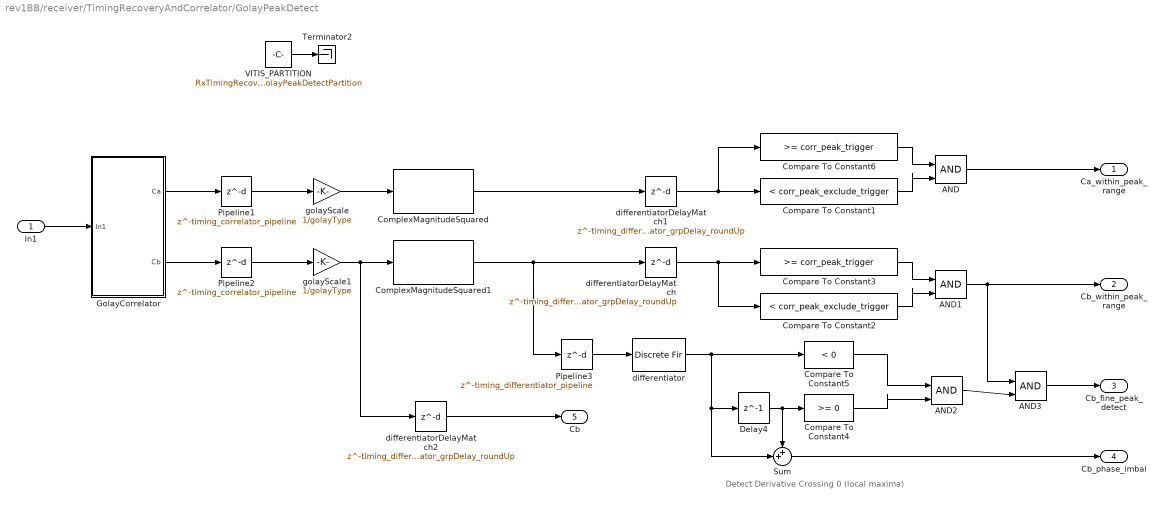
== system rev1BB/receiver/TimingRecoveryAndCorrelator/GolayPeakDetect ==
  note: Detect Derivative Crossing 0 (local maxima)
  In1 : Inport
  AND{,1..3} (4 alike) : Logic  IconShape=distinctive  AllPortsSameDT=off  OutDataTypeStr=boolean
  Compare To Constant1 : simulink/Logic and Bit Operations/Compare To Constant  relop=<  const=corr_peak_exclude_trigger  OutDataTypeStr=boolean
  Compare To Constant2 : simulink/Logic and Bit Operations/Compare To Constant  relop=<  const=corr_peak_exclude_trigger  OutDataTypeStr=boolean
  Compare To Constant3 : simulink/Logic and Bit Operations/Compare To Constant  relop=>=  const=corr_peak_trigger  OutDataTypeStr=boolean
  Compare To Constant4 : simulink/Logic and Bit Operations/Compare To Constant  relop=>=  const=0  OutDataTypeStr=boolean
  Compare To Constant5 : simulink/Logic and Bit Operations/Compare To Constant  relop=<  const=0  OutDataTypeStr=boolean
  Compare To Constant6 : simulink/Logic and Bit Operations/Compare To Constant  relop=>=  const=corr_peak_trigger  OutDataTypeStr=boolean
  ComplexMagnitudeSquared : rev1CyclopsLib/ComplexMagnitudeSquared  SystemSampleTime=-1  VariantActivationTime=update diagram  Latency=0  AutoFrameSizeCalculation=off
  ComplexMagnitudeSquared1 : rev1CyclopsLib/ComplexMagnitudeSquared  SystemSampleTime=-1  VariantActivationTime=update diagram  Latency=0  AutoFrameSizeCalculation=off
  Delay4 : Delay  DelayLength=1
  GolayCorrelator : Subsystem
  Pipeline1 : Delay  DelayLength=timing_correlator_pipeline
  Pipeline2 : Delay  DelayLength=timing_correlator_pipeline
  Pipeline3 : Delay  DelayLength=timing_differentiator_pipeline
  Sum : Sum  Inputs=++|  OutDataTypeStr=Inherit: Same as first input
  Terminator2 : Terminator
  VITIS_PARTITION : Constant  Value=RxTimingRecoveryGolayPeakDetectPartition
  differentiator : DiscreteFir  Coefficients=timingDifferentiatorFilt
  differentiatorDelayMatch : Delay  DelayLength=timing_differentiator_grpDelay_roundUp
  differentiatorDelayMatch1 : Delay  DelayLength=timing_differentiator_grpDelay_roundUp
  differentiatorDelayMatch2 : Delay  DelayLength=timing_differentiator_grpDelay_roundUp
  golayScale : Gain  Gain=1/golayType
  golayScale1 : Gain  Gain=1/golayType
  Ca_within_peak_range : Outport
  Cb_within_peak_range : Outport  Port=2
  Cb_fine_peak_detect : Outport  Port=3
  Cb_phase_imbal : Outport  Port=4
  Cb : Outport  Port=5
  wires:
  AND/1 -> Ca_within_peak_range/1
  Compare To Constant1/1 -> AND/2
  Compare To Constant6/1 -> AND/1
  differentiatorDelayMatch/1 -> Compare To Constant2/1, Compare To Constant3/1
  golayScale1/1 -> ComplexMagnitudeSquared1/1, differentiatorDelayMatch2/1
  Compare To Constant2/1 -> AND1/2
  AND1/1 -> AND3/1, Cb_within_peak_range/1
  differentiatorDelayMatch1/1 -> Compare To Constant6/1, Compare To Constant1/1
  golayScale/1 -> ComplexMagnitudeSquared/1
  Compare To Constant3/1 -> AND1/1
  Delay4/1 -> Sum/1, Compare To Constant4/1
  differentiator/1 -> Compare To Constant5/1, Sum/2, Delay4/1
  Compare To Constant5/1 -> AND2/1
  Compare To Constant4/1 -> AND2/2
  AND2/1 -> AND3/2
  AND3/1 -> Cb_fine_peak_detect/1
  Sum/1 -> Cb_phase_imbal/1
  VITIS_PARTITION/1 -> Terminator2/1
  In1/1 -> GolayCorrelator/1(In1)
  GolayCorrelator/1(Ca) -> Pipeline1/1
  GolayCorrelator/2(Cb) -> Pipeline2/1
  ComplexMagnitudeSquared/1 -> differentiatorDelayMatch1/1
  ComplexMagnitudeSquared1/1 -> differentiatorDelayMatch/1, Pipeline3/1
  differentiatorDelayMatch2/1 -> Cb/1
  Pipeline3/1 -> differentiator/1
  Pipeline1/1 -> golayScale/1
  Pipeline2/1 -> golayScale1/1

== system rev1BB/receiver/TimingRecoveryAndCorrelator/GolayPeakDetectDecimSync ==
  In1 : Inport
  In2 : Inport  Port=2
  Cb : Inport  Port=3
  idx : Inport  Port=4
  Selector1 : Selector  IndexMode=Zero-based  InputPortWidth=overSample  IndexOptions=Index vector (port)  Indices=[1 3]  OutputSizes=1
  Selector2 : Selector  IndexMode=Zero-based  InputPortWidth=overSample  IndexOptions=Index vector (port)  Indices=[1 3]  OutputSizes=1
  Selector3 : Selector  IndexMode=Zero-based  InputPortWidth=overSample  IndexOptions=Index vector (port)  Indices=[1 3]  OutputSizes=1
  Tapped Delay1 : simulink/Discrete/Tapped Delay  vinit=0.0  samptime=-1  NumDelays=overSample-1  DelayOrder=Newest  includeCurrent=on
  Tapped Delay2 : simulink/Discrete/Tapped Delay  vinit=0.0  samptime=-1  NumDelays=overSample-1  DelayOrder=Newest  includeCurrent=on
  Tapped Delay3 : simulink/Discrete/Tapped Delay  vinit=0.0  samptime=-1  NumDelays=overSample-1  DelayOrder=Newest  includeCurrent=on
  Terminator2 : Terminator
  VITIS_PARTITION : Constant  Value=RxTimingRecoverySymbolClockPartition
  Out1 : Outport
  Out2 : Outport  Port=2
  Out3 : Outport  Port=3
  wires:
  Tapped Delay2/1 -> Selector2/1
  Tapped Delay3/1 -> Selector3/1
  Selector2/1 -> Out1/1
  Selector3/1 -> Out2/1
  Selector1/1 -> Out3/1
  Tapped Delay1/1 -> Selector1/1
  idx/1 -> Selector1/2, Selector3/2, Selector2/2
  In1/1 -> Tapped Delay2/1
  In2/1 -> Tapped Delay3/1
  Cb/1 -> Tapped Delay1/1
  VITIS_PARTITION/1 -> Terminator2/1

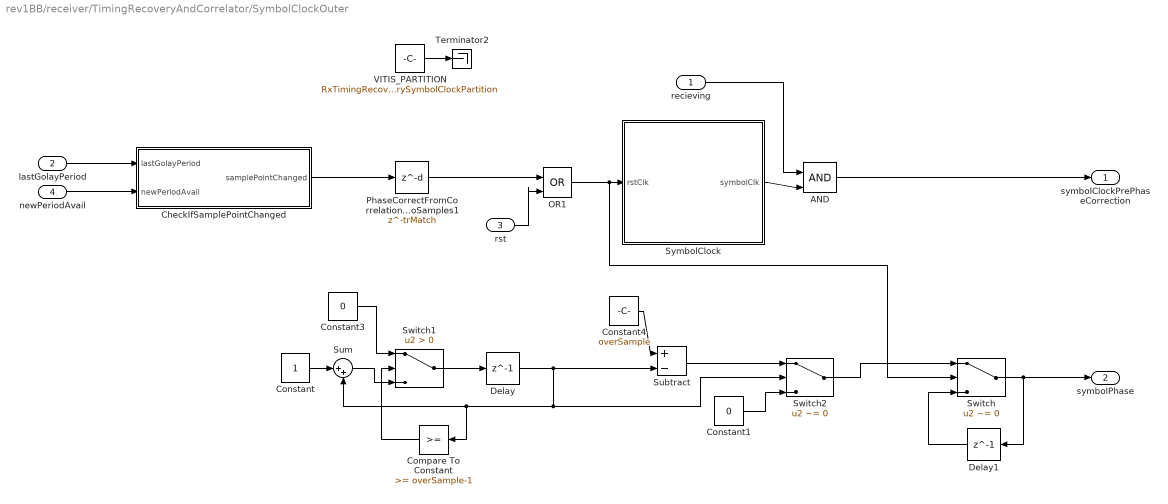
== system rev1BB/receiver/TimingRecoveryAndCorrelator/SymbolClockOuter ==
  recieving : Inport
  lastGolayPeriod : Inport  Port=2
  rst : Inport  Port=3
  newPeriodAvail : Inport  Port=4
  AND : Logic  IconShape=distinctive  AllPortsSameDT=off  OutDataTypeStr=boolean
  CheckIfSamplePointChanged : Subsystem
  Compare To Constant : simulink/Logic and Bit Operations/Compare To Constant  relop=>=  const=overSample-1  OutDataTypeStr=boolean
  Constant : Constant  OutDataTypeStr=uint8
  Constant1 : Constant  Value=0  OutDataTypeStr=uint8
  Constant3 : Constant  Value=0  OutDataTypeStr=uint8
  Constant4 : Constant  Value=overSample  OutDataTypeStr=uint8
  Delay : Delay  DelayLength=1  InitialCondition=trIntPhaseCounterInit
  Delay1 : Delay  DelayLength=1
  OR1 : Logic  Operator=OR  IconShape=distinctive  AllPortsSameDT=off  OutDataTypeStr=boolean
  PhaseCorrectFromCorrelationToSamples1 : Delay  DelayLength=trMatch
  Subtract : Sum  Inputs=+-
  Sum : Sum  Inputs=|++
  Switch : Switch  Criteria=u2 ~= 0
  Switch1 : Switch  Criteria=u2 > Threshold
  Switch2 : Switch  Criteria=u2 ~= 0
  SymbolClock : Subsystem
  Terminator2 : Terminator
  VITIS_PARTITION : Constant  Value=RxTimingRecoverySymbolClockPartition
  symbolClockPrePhaseCorrection : Outport
  symbolPhase : Outport  Port=2
  wires:
  lastGolayPeriod/1 -> CheckIfSamplePointChanged/1(lastGolayPeriod)
  SymbolClock/1(symbolClk) -> AND/2
  CheckIfSamplePointChanged/1(samplePointChanged) -> PhaseCorrectFromCorrelationToSamples1/1
  newPeriodAvail/1 -> CheckIfSamplePointChanged/2(newPeriodAvail)
  recieving/1 -> AND/1
  rst/1 -> OR1/2
  PhaseCorrectFromCorrelationToSamples1/1 -> OR1/1
  AND/1 -> symbolClockPrePhaseCorrection/1
  OR1/1 -> Switch/2, SymbolClock/1(rstClk)
  VITIS_PARTITION/1 -> Terminator2/1
  Constant/1 -> Sum/1
  Delay1/1 -> Switch/3
  Switch1/1 -> Delay/1
  Sum/1 -> Switch1/3
  Constant3/1 -> Switch1/1
  Compare To Constant/1 -> Switch1/2
  Constant4/1 -> Subtract/1
  Subtract/1 -> Switch2/1
  Switch/1 -> symbolPhase/1, Delay1/1
  Delay/1 -> Subtract/2, Compare To Constant/1, Sum/2, Switch2/2
  Constant1/1 -> Switch2/3
  Switch2/1 -> Switch/1

== system rev1BB/receiver/TimingRecoveryAndCorrelator/TRControl ==
  cef_start : Inport
  peak : Inport  Port=2
  rst : Inport  Port=3
  PhaseCorrectFromCorrelationToSamples : Delay  DelayLength=trMatch
  Terminator : Terminator
  Terminator2 : Terminator
  VITIS_PARTITION : Constant  Value=RxTimingRecoveryControlPartition
  edgeDetect : Subsystem
  tr_control : Stateflow chart  TreatAsAtomicUnit=on
  receiving : Outport
  lastPeriod : Outport  Port=2
  rstIntegerPhase : Outport  Port=3
  estimateNow : Outport  Port=4
  trEstDoneEdge : Outport  Port=5
  trEstDone : Outport  Port=6
  wires:
  PhaseCorrectFromCorrelationToSamples/1 -> rstIntegerPhase/1
  tr_control/6(lastPeriod) -> lastPeriod/1
  tr_control/1(resetIntegerPhase) -> PhaseCorrectFromCorrelationToSamples/1
  peak/1 -> tr_control/1(peak)
  edgeDetect/1(rst) -> trEstDoneEdge/1
  rst/1 -> tr_control/2(rst)
  tr_control/4(estimateNow) -> estimateNow/1
  cef_start/1 -> tr_control/3(cef_start)
  tr_control/3(estimateOK) -> Terminator/1
  tr_control/2(receiving) -> receiving/1
  tr_control/5(trEstDone) -> edgeDetect/1(In1), trEstDone/1
  VITIS_PARTITION/1 -> Terminator2/1

== system rev1BB/receiver/TimingRecoveryAndCorrelator/VarDelayDecimSync ==
  idx : Inport
  In2 : Inport  Port=2
  Selector : Selector  IndexMode=Zero-based  InputPortWidth=overSample  IndexOptions=Index vector (port)  Indices=[1 3]  OutputSizes=1
  Tapped Delay : simulink/Discrete/Tapped Delay  vinit=0.0  samptime=-1  NumDelays=overSample-1  DelayOrder=Newest  includeCurrent=on
  Terminator2 : Terminator
  VITIS_PARTITION : Constant  Value=RxTimingRecoverySymbolClockPartition
  Out1 : Outport
  wires:
  Selector/1 -> Out1/1
  Tapped Delay/1 -> Selector/1
  idx/1 -> Selector/2
  In2/1 -> Tapped Delay/1
  VITIS_PARTITION/1 -> Terminator2/1

== system rev1BB/receiver/TimingRecoveryAndCorrelator/VarDelayWithSampleAlignment ==
  samples : Inport
  delay : Inport  Port=2
  AlignSymbolWithCorrelatorOutput2 : Delay  DelayLength=timing_differentiator_grpDelay_roundUp  UseCircularBuffer=on
  Terminator2 : Terminator
  TimingDelayVal : Scope
  VITIS_PARTITION : Constant  Value=RxTimingRecoveryVariableDelayPartition
  VarDelay : Subsystem  AncestorBlock=rev1CyclopsLib/VarDelay
  out : Outport
  Out2 : Outport  Port=2
  wires:
  AlignSymbolWithCorrelatorOutput2/1 -> Out2/1
  samples/1 -> VarDelay/1(samples)
  VarDelay/1(out) -> out/1, AlignSymbolWithCorrelatorOutput2/1
  VITIS_PARTITION/1 -> Terminator2/1
  delay/1 -> TimingDelayVal/1, VarDelay/2(delay)

== system rev1BB/transmitter_outer/transmitter/VITIS_CLOCK_DOMAIN_modulate ==
  symbol : Inport
  modulation : Inport  Port=2
  en : Inport  Port=3
  ClockDomainDummy_Bugfix : Delay  DelayLength=0
  Upsample : dspsigops/Upsample  N=overSample  phase=0  RateOptions=Allow multirate processing  ic=0  mode=Unused parameter value
  Upsample2 : dspsigops/Upsample  N=overSample  phase=0  RateOptions=Allow multirate processing  ic=0  mode=Unused parameter value
  modulator : Subsystem
  symbolUpsampled : Outport
  enUpsampled : Outport  Port=2
  wires:
  symbol/1 -> modulator/1(symbols)
  Upsample/1 -> symbolUpsampled/1
  modulation/1 -> modulator/2(modulationMode)
  Upsample2/1 -> enUpsampled/1
  modulator/1(modulatedSymbols) -> Upsample/1
  en/1 -> ClockDomainDummy_Bugfix/1
  ClockDomainDummy_Bugfix/1 -> Upsample2/1

== system rev1BB/transmitter_outer/transmitter/rootRaisedCosineAndScale ==
  note: The additional scale factor in the RRC filter is due to the zero filling (upsample by 4) and allows us to output 0 dB power (relative to 1 Ohm) at the output of the filter.
  In1 : Inport
  Terminator2 : Terminator
  VITIS_PARTITION : Constant  Value=TxRRCFilterPartition
  rootRaisedCosineFilter : DiscreteFir  Coefficients=rcTxFilt.*sqrt(overSample)
  Out1 : Outport
  wires:
  rootRaisedCosineFilter/1 -> Out1/1
  In1/1 -> rootRaisedCosineFilter/1
  VITIS_PARTITION/1 -> Terminator2/1

== system rev1BB/receiver/AGC/AGCLoopAndCorrect/AGCCorrectionLoopEnabled ==
  note: Adapted to be closer to the Log AGC used in matlab which scales the detected signal in the loop (rather than scaling the input). This is OK because we are using floating point and therefore do not need to worry about loss of resolution in the detector / filter.
  samples : Inport
  Enable : EnablePort
  AccumulatorWithSaturationCombinationalOutput : rev1CyclopsLib/AccumulatorWithSaturationCombinationalOutput  SatUp=agc_sat_up  SatDown=agc_sat_low
  Constant : Constant  Value=agcDesired  OutDataTypeStr=Inherit: Inherit via back propagation
  Exp : Math  SaturateOnIntegerOverflow=on
  Gain : Gain  Gain=agcStep
  Pipeline{,1..3} (4 alike) : Delay  DelayLength=1
  Product1 : Product  OutDataTypeStr=Inherit: Same as first input
  Product2 : Product  OutDataTypeStr=Inherit: Same as first input
  Sum1 : Sum  Inputs=|-+
  Terminator : Terminator
  ln : Math  Operator=log  SaturateOnIntegerOverflow=on
  correction : Outport
  lnPwr : Outport  Port=2
  wires:
  Product1/1 -> Pipeline1/1
  Product2/1 -> Product1/2
  Sum1/1 -> Gain/1
  Gain/1 -> AccumulatorWithSaturationCombinationalOutput/1
  ln/1 -> Pipeline/1
  Exp/1 -> Pipeline2/1
  samples/1 -> Product1/1
  Constant/1 -> Sum1/2
  AccumulatorWithSaturationCombinationalOutput/2 -> Pipeline3/1
  AccumulatorWithSaturationCombinationalOutput/1 -> Terminator/1
  Pipeline/1 -> lnPwr/1, Sum1/1
  Pipeline1/1 -> ln/1
  Pipeline2/1 -> correction/1, Product2/2, Product2/1
  Pipeline3/1 -> Exp/1

== system rev1BB/receiver/AGC/AGCPwrAvg/AGCPowerAvgEnabled ==
  samples : Inport
  Enable : EnablePort
  ComplexMagnitudeSquared : rev1CyclopsLib/ComplexMagnitudeSquared  SystemSampleTime=-1  VariantActivationTime=update diagram  Latency=0  AutoFrameSizeCalculation=off
  RollingAverage : rev1CyclopsLib/RollingAverage  averagingSamples=agc_detector_taps
  lnPwrAvg : Outport
  wires:
  samples/1 -> ComplexMagnitudeSquared/1
  RollingAverage/1 -> lnPwrAvg/1
  ComplexMagnitudeSquared/1 -> RollingAverage/1

== system rev1BB/receiver/SymbolDomainOuter/VITIS_CLOCK_DOMAIN_SymbolDomain/CoarseCFOCorrect ==
  symbolIn : Inport
  Cb_within_peak_range : Inport  Port=2
  Cb : Inport  Port=3
  inSTF : Inport  Port=4
  inCEF : Inport  Port=5
  rst : Inport  Port=6
  ApplyCorrection : Subsystem
  CoarseCFOEstimate : Subsystem
  Terminator2 : Terminator
  VITIS_PARTITION : Constant  Value=RxCoarseCFOPartition
  symbolOut : Outport
  wires:
  Cb_within_peak_range/1 -> CoarseCFOEstimate/1(correlationPeak)
  Cb/1 -> CoarseCFOEstimate/2(correlation)
  inSTF/1 -> CoarseCFOEstimate/3(inSTF)
  inCEF/1 -> CoarseCFOEstimate/4(inCEF)
  rst/1 -> CoarseCFOEstimate/5(rst)
  ApplyCorrection/1(symbolOut) -> symbolOut/1
  symbolIn/1 -> ApplyCorrection/2(symbolIn)
  CoarseCFOEstimate/1(phaseIncrement) -> ApplyCorrection/1(phaseIncrement)
  VITIS_PARTITION/1 -> Terminator2/1

== system rev1BB/receiver/SymbolDomainOuter/VITIS_CLOCK_DOMAIN_SymbolDomain/DataPacker ==
  demodSymbol : Inport
  modulationType : Inport  Port=2
  inPayload : Inport  Port=3
  inHeader : Inport  Port=4
  dataLast : Inport  Port=5
  rst : Inport  Port=6
  " BitsPerSymbol 1-D Lookup Table" : Lookup_n-D  NumberOfTableDimensions=1  BreakpointsForDimension1=modKeys  IndexSearchMethod=Evenly spaced points  Table=modBPS  InterpMethod=Flat  DiagnosticForOutOfRangeInput=Error  InternalRulePriority=Speed  RndMeth=Simplest  InputSameDT=on
  Saturation : Saturate  UpperLimit=modKeys(length(modKeys))  LowerLimit=modKeys(1)
  Terminator : Terminator
  Terminator1 : Terminator
  Terminator2 : Terminator
  VITIS_PARTITION : Constant  Value=RxPackerPartition
  dataPacker : Stateflow chart  TreatAsAtomicUnit=on
  dataPacked : Outport
  dataPackedValid : Outport  Port=2
  dataPackedLast : Outport  Port=3
  wires:
  VITIS_PARTITION/1 -> Terminator2/1
  demodSymbol/1 -> dataPacker/4(data)
  dataPacker/2(packed_data) -> dataPacked/1
  dataPacker/3(valid) -> dataPackedValid/1
  dataPacker/1(last_out) -> dataPackedLast/1
  dataPacker/4(decoding) -> Terminator/1
  dataPacker/5(err) -> Terminator1/1
  " BitsPerSymbol 1-D Lookup Table"/1 -> dataPacker/3(bitsPerSymbolMod)
  Saturation/1 -> " BitsPerSymbol 1-D Lookup Table"/1
  modulationType/1 -> Saturation/1
  inPayload/1 -> dataPacker/5(payload)
  inHeader/1 -> dataPacker/2(header)
  dataLast/1 -> dataPacker/1(last_in)
  rst/1 -> dataPacker/6(rst)

== system rev1BB/receiver/SymbolDomainOuter/VITIS_CLOCK_DOMAIN_SymbolDomain/DelayMatchForEq ==
  rst : Inport
  cefDoneEarlyWarning : Inport  Port=2
  rstFineCFO : Inport  Port=3
  dataValid : Inport  Port=4
  dataLast : Inport  Port=5
  DelayMatchForEq{,1..4} (5 alike) : Delay  DelayLength=lmsEqDepth/2-1  UseCircularBuffer=on
  Terminator2 : Terminator
  VITIS_PARTITION : Constant  Value=RxPacketControllerPartition
  rstOut : Outport
  cefDoneEarlyWarningOut : Outport  Port=2
  rstFineCFOOut : Outport  Port=3
  dataValidOut : Outport  Port=4
  dataLastOut : Outport  Port=5
  wires:
  DelayMatchForEq3/1 -> dataLastOut/1
  DelayMatchForEq/1 -> cefDoneEarlyWarningOut/1
  dataLast/1 -> DelayMatchForEq3/1
  rstFineCFO/1 -> DelayMatchForEq1/1
  cefDoneEarlyWarning/1 -> DelayMatchForEq/1
  dataValid/1 -> DelayMatchForEq2/1
  DelayMatchForEq2/1 -> dataValidOut/1
  DelayMatchForEq1/1 -> rstFineCFOOut/1
  VITIS_PARTITION/1 -> Terminator2/1
  DelayMatchForEq4/1 -> rstOut/1
  rst/1 -> DelayMatchForEq4/1

== system rev1BB/receiver/SymbolDomainOuter/VITIS_CLOCK_DOMAIN_SymbolDomain/DelayMatchForEq1 ==
  freezeCFO : Inport
  DelayMatchForEq : Delay  DelayLength=lmsEqDepth/2-1  UseCircularBuffer=on
  Terminator2 : Terminator
  VITIS_PARTITION : Constant  Value=RxPacketControllerPartition
  freezeCFOOut : Outport
  wires:
  DelayMatchForEq/1 -> freezeCFOOut/1
  freezeCFO/1 -> DelayMatchForEq/1
  VITIS_PARTITION/1 -> Terminator2/1
